simulink model "gm_parallel_lht"  (R2019b)
settings: Solver=FixedStepDiscrete  StartTime=0.0  StopTime=inf  RelTol=1e-3
undefined symbols (not defined in the file or in its folder): bt, height, width
libraries: hdlsllib x190, simulink x13, hdlmdlgenlib x7, dspsrcs4 x1
(part 14 of 18)

== system gm_parallel_lht/Parallel LHT/Parallel LHT Accumulator/Accumulator with Switches/Accumulator_instance150/Block RAM/Simple Dual Port RAM ==
  wr_data : Inport  OutDataTypeStr=fixdt(0, 11, 0)  PortDimensions=1  SampleTime=6.66666666666667e-09
  wr_addr : Inport  Port=2  OutDataTypeStr=fixdt(0, 11, 0)  PortDimensions=1  SampleTime=6.66666666666667e-09
  wr_en : Inport  Port=3  OutDataTypeStr=boolean  PortDimensions=1  SampleTime=6.66666666666667e-09
  rd_addr : Inport  Port=4  OutDataTypeStr=fixdt(0, 11, 0)  PortDimensions=1  SampleTime=6.66666666666667e-09
  Simple Dual Port RAM : hdlsllib/HDL RAMs/Simple Dual Port RAM  ram_size=ceil(log2(maxRho*2))
      settings: SourceProductName=Simulink  SourceProductBaseCode=SL
  rd_data : Outport
  wires:
  rd_addr/1 -> Simple Dual Port RAM/4
  wr_en/1 -> Simple Dual Port RAM/3
  wr_addr/1 -> Simple Dual Port RAM/2
  wr_data/1 -> Simple Dual Port RAM/1
  Simple Dual Port RAM/1 -> rd_data/1

== system gm_parallel_lht/Parallel LHT/Parallel LHT Accumulator/Accumulator with Switches/Accumulator_instance151/Block RAM/Simple Dual Port RAM ==
  wr_data : Inport  OutDataTypeStr=fixdt(0, 11, 0)  PortDimensions=1  SampleTime=6.66666666666667e-09
  wr_addr : Inport  Port=2  OutDataTypeStr=fixdt(0, 11, 0)  PortDimensions=1  SampleTime=6.66666666666667e-09
  wr_en : Inport  Port=3  OutDataTypeStr=boolean  PortDimensions=1  SampleTime=6.66666666666667e-09
  rd_addr : Inport  Port=4  OutDataTypeStr=fixdt(0, 11, 0)  PortDimensions=1  SampleTime=6.66666666666667e-09
  Simple Dual Port RAM : hdlsllib/HDL RAMs/Simple Dual Port RAM  ram_size=ceil(log2(maxRho*2))
      settings: SourceProductName=Simulink  SourceProductBaseCode=SL
  rd_data : Outport
  wires:
  rd_addr/1 -> Simple Dual Port RAM/4
  wr_en/1 -> Simple Dual Port RAM/3
  wr_addr/1 -> Simple Dual Port RAM/2
  wr_data/1 -> Simple Dual Port RAM/1
  Simple Dual Port RAM/1 -> rd_data/1

== system gm_parallel_lht/Parallel LHT/Parallel LHT Accumulator/Accumulator with Switches/Accumulator_instance152/Block RAM/Simple Dual Port RAM ==
  wr_data : Inport  OutDataTypeStr=fixdt(0, 11, 0)  PortDimensions=1  SampleTime=6.66666666666667e-09
  wr_addr : Inport  Port=2  OutDataTypeStr=fixdt(0, 11, 0)  PortDimensions=1  SampleTime=6.66666666666667e-09
  wr_en : Inport  Port=3  OutDataTypeStr=boolean  PortDimensions=1  SampleTime=6.66666666666667e-09
  rd_addr : Inport  Port=4  OutDataTypeStr=fixdt(0, 11, 0)  PortDimensions=1  SampleTime=6.66666666666667e-09
  Simple Dual Port RAM : hdlsllib/HDL RAMs/Simple Dual Port RAM  ram_size=ceil(log2(maxRho*2))
      settings: SourceProductName=Simulink  SourceProductBaseCode=SL
  rd_data : Outport
  wires:
  rd_addr/1 -> Simple Dual Port RAM/4
  wr_en/1 -> Simple Dual Port RAM/3
  wr_addr/1 -> Simple Dual Port RAM/2
  wr_data/1 -> Simple Dual Port RAM/1
  Simple Dual Port RAM/1 -> rd_data/1

== system gm_parallel_lht/Parallel LHT/Parallel LHT Accumulator/Accumulator with Switches/Accumulator_instance153/Block RAM/Simple Dual Port RAM ==
  wr_data : Inport  OutDataTypeStr=fixdt(0, 11, 0)  PortDimensions=1  SampleTime=6.66666666666667e-09
  wr_addr : Inport  Port=2  OutDataTypeStr=fixdt(0, 11, 0)  PortDimensions=1  SampleTime=6.66666666666667e-09
  wr_en : Inport  Port=3  OutDataTypeStr=boolean  PortDimensions=1  SampleTime=6.66666666666667e-09
  rd_addr : Inport  Port=4  OutDataTypeStr=fixdt(0, 11, 0)  PortDimensions=1  SampleTime=6.66666666666667e-09
  Simple Dual Port RAM : hdlsllib/HDL RAMs/Simple Dual Port RAM  ram_size=ceil(log2(maxRho*2))
      settings: SourceProductName=Simulink  SourceProductBaseCode=SL
  rd_data : Outport
  wires:
  rd_addr/1 -> Simple Dual Port RAM/4
  wr_en/1 -> Simple Dual Port RAM/3
  wr_addr/1 -> Simple Dual Port RAM/2
  wr_data/1 -> Simple Dual Port RAM/1
  Simple Dual Port RAM/1 -> rd_data/1

== system gm_parallel_lht/Parallel LHT/Parallel LHT Accumulator/Accumulator with Switches/Accumulator_instance154/Block RAM/Simple Dual Port RAM ==
  wr_data : Inport  OutDataTypeStr=fixdt(0, 11, 0)  PortDimensions=1  SampleTime=6.66666666666667e-09
  wr_addr : Inport  Port=2  OutDataTypeStr=fixdt(0, 11, 0)  PortDimensions=1  SampleTime=6.66666666666667e-09
  wr_en : Inport  Port=3  OutDataTypeStr=boolean  PortDimensions=1  SampleTime=6.66666666666667e-09
  rd_addr : Inport  Port=4  OutDataTypeStr=fixdt(0, 11, 0)  PortDimensions=1  SampleTime=6.66666666666667e-09
  Simple Dual Port RAM : hdlsllib/HDL RAMs/Simple Dual Port RAM  ram_size=ceil(log2(maxRho*2))
      settings: SourceProductName=Simulink  SourceProductBaseCode=SL
  rd_data : Outport
  wires:
  rd_addr/1 -> Simple Dual Port RAM/4
  wr_en/1 -> Simple Dual Port RAM/3
  wr_addr/1 -> Simple Dual Port RAM/2
  wr_data/1 -> Simple Dual Port RAM/1
  Simple Dual Port RAM/1 -> rd_data/1

== system gm_parallel_lht/Parallel LHT/Parallel LHT Accumulator/Accumulator with Switches/Accumulator_instance155/Block RAM/Simple Dual Port RAM ==
  wr_data : Inport  OutDataTypeStr=fixdt(0, 11, 0)  PortDimensions=1  SampleTime=6.66666666666667e-09
  wr_addr : Inport  Port=2  OutDataTypeStr=fixdt(0, 11, 0)  PortDimensions=1  SampleTime=6.66666666666667e-09
  wr_en : Inport  Port=3  OutDataTypeStr=boolean  PortDimensions=1  SampleTime=6.66666666666667e-09
  rd_addr : Inport  Port=4  OutDataTypeStr=fixdt(0, 11, 0)  PortDimensions=1  SampleTime=6.66666666666667e-09
  Simple Dual Port RAM : hdlsllib/HDL RAMs/Simple Dual Port RAM  ram_size=ceil(log2(maxRho*2))
      settings: SourceProductName=Simulink  SourceProductBaseCode=SL
  rd_data : Outport
  wires:
  rd_addr/1 -> Simple Dual Port RAM/4
  wr_en/1 -> Simple Dual Port RAM/3
  wr_addr/1 -> Simple Dual Port RAM/2
  wr_data/1 -> Simple Dual Port RAM/1
  Simple Dual Port RAM/1 -> rd_data/1

== system gm_parallel_lht/Parallel LHT/Parallel LHT Accumulator/Accumulator with Switches/Accumulator_instance156/Block RAM/Simple Dual Port RAM ==
  wr_data : Inport  OutDataTypeStr=fixdt(0, 11, 0)  PortDimensions=1  SampleTime=6.66666666666667e-09
  wr_addr : Inport  Port=2  OutDataTypeStr=fixdt(0, 11, 0)  PortDimensions=1  SampleTime=6.66666666666667e-09
  wr_en : Inport  Port=3  OutDataTypeStr=boolean  PortDimensions=1  SampleTime=6.66666666666667e-09
  rd_addr : Inport  Port=4  OutDataTypeStr=fixdt(0, 11, 0)  PortDimensions=1  SampleTime=6.66666666666667e-09
  Simple Dual Port RAM : hdlsllib/HDL RAMs/Simple Dual Port RAM  ram_size=ceil(log2(maxRho*2))
      settings: SourceProductName=Simulink  SourceProductBaseCode=SL
  rd_data : Outport
  wires:
  rd_addr/1 -> Simple Dual Port RAM/4
  wr_en/1 -> Simple Dual Port RAM/3
  wr_addr/1 -> Simple Dual Port RAM/2
  wr_data/1 -> Simple Dual Port RAM/1
  Simple Dual Port RAM/1 -> rd_data/1

== system gm_parallel_lht/Parallel LHT/Parallel LHT Accumulator/Accumulator with Switches/Accumulator_instance157/Block RAM/Simple Dual Port RAM ==
  wr_data : Inport  OutDataTypeStr=fixdt(0, 11, 0)  PortDimensions=1  SampleTime=6.66666666666667e-09
  wr_addr : Inport  Port=2  OutDataTypeStr=fixdt(0, 11, 0)  PortDimensions=1  SampleTime=6.66666666666667e-09
  wr_en : Inport  Port=3  OutDataTypeStr=boolean  PortDimensions=1  SampleTime=6.66666666666667e-09
  rd_addr : Inport  Port=4  OutDataTypeStr=fixdt(0, 11, 0)  PortDimensions=1  SampleTime=6.66666666666667e-09
  Simple Dual Port RAM : hdlsllib/HDL RAMs/Simple Dual Port RAM  ram_size=ceil(log2(maxRho*2))
      settings: SourceProductName=Simulink  SourceProductBaseCode=SL
  rd_data : Outport
  wires:
  rd_addr/1 -> Simple Dual Port RAM/4
  wr_en/1 -> Simple Dual Port RAM/3
  wr_addr/1 -> Simple Dual Port RAM/2
  wr_data/1 -> Simple Dual Port RAM/1
  Simple Dual Port RAM/1 -> rd_data/1

== system gm_parallel_lht/Parallel LHT/Parallel LHT Accumulator/Accumulator with Switches/Accumulator_instance158/Block RAM/Simple Dual Port RAM ==
  wr_data : Inport  OutDataTypeStr=fixdt(0, 11, 0)  PortDimensions=1  SampleTime=6.66666666666667e-09
  wr_addr : Inport  Port=2  OutDataTypeStr=fixdt(0, 11, 0)  PortDimensions=1  SampleTime=6.66666666666667e-09
  wr_en : Inport  Port=3  OutDataTypeStr=boolean  PortDimensions=1  SampleTime=6.66666666666667e-09
  rd_addr : Inport  Port=4  OutDataTypeStr=fixdt(0, 11, 0)  PortDimensions=1  SampleTime=6.66666666666667e-09
  Simple Dual Port RAM : hdlsllib/HDL RAMs/Simple Dual Port RAM  ram_size=ceil(log2(maxRho*2))
      settings: SourceProductName=Simulink  SourceProductBaseCode=SL
  rd_data : Outport
  wires:
  rd_addr/1 -> Simple Dual Port RAM/4
  wr_en/1 -> Simple Dual Port RAM/3
  wr_addr/1 -> Simple Dual Port RAM/2
  wr_data/1 -> Simple Dual Port RAM/1
  Simple Dual Port RAM/1 -> rd_data/1

== system gm_parallel_lht/Parallel LHT/Parallel LHT Accumulator/Accumulator with Switches/Accumulator_instance159/Block RAM/Simple Dual Port RAM ==
  wr_data : Inport  OutDataTypeStr=fixdt(0, 11, 0)  PortDimensions=1  SampleTime=6.66666666666667e-09
  wr_addr : Inport  Port=2  OutDataTypeStr=fixdt(0, 11, 0)  PortDimensions=1  SampleTime=6.66666666666667e-09
  wr_en : Inport  Port=3  OutDataTypeStr=boolean  PortDimensions=1  SampleTime=6.66666666666667e-09
  rd_addr : Inport  Port=4  OutDataTypeStr=fixdt(0, 11, 0)  PortDimensions=1  SampleTime=6.66666666666667e-09
  Simple Dual Port RAM : hdlsllib/HDL RAMs/Simple Dual Port RAM  ram_size=ceil(log2(maxRho*2))
      settings: SourceProductName=Simulink  SourceProductBaseCode=SL
  rd_data : Outport
  wires:
  rd_addr/1 -> Simple Dual Port RAM/4
  wr_en/1 -> Simple Dual Port RAM/3
  wr_addr/1 -> Simple Dual Port RAM/2
  wr_data/1 -> Simple Dual Port RAM/1
  Simple Dual Port RAM/1 -> rd_data/1

== system gm_parallel_lht/Parallel LHT/Parallel LHT Accumulator/Accumulator with Switches/Accumulator_instance16/Block RAM/Simple Dual Port RAM ==
  wr_data : Inport  OutDataTypeStr=fixdt(0, 11, 0)  PortDimensions=1  SampleTime=6.66666666666667e-09
  wr_addr : Inport  Port=2  OutDataTypeStr=fixdt(0, 11, 0)  PortDimensions=1  SampleTime=6.66666666666667e-09
  wr_en : Inport  Port=3  OutDataTypeStr=boolean  PortDimensions=1  SampleTime=6.66666666666667e-09
  rd_addr : Inport  Port=4  OutDataTypeStr=fixdt(0, 11, 0)  PortDimensions=1  SampleTime=6.66666666666667e-09
  Simple Dual Port RAM : hdlsllib/HDL RAMs/Simple Dual Port RAM  ram_size=ceil(log2(maxRho*2))
      settings: SourceProductName=Simulink  SourceProductBaseCode=SL
  rd_data : Outport
  wires:
  rd_addr/1 -> Simple Dual Port RAM/4
  wr_en/1 -> Simple Dual Port RAM/3
  wr_addr/1 -> Simple Dual Port RAM/2
  wr_data/1 -> Simple Dual Port RAM/1
  Simple Dual Port RAM/1 -> rd_data/1

== system gm_parallel_lht/Parallel LHT/Parallel LHT Accumulator/Accumulator with Switches/Accumulator_instance160/Block RAM/Simple Dual Port RAM ==
  wr_data : Inport  OutDataTypeStr=fixdt(0, 11, 0)  PortDimensions=1  SampleTime=6.66666666666667e-09
  wr_addr : Inport  Port=2  OutDataTypeStr=fixdt(0, 11, 0)  PortDimensions=1  SampleTime=6.66666666666667e-09
  wr_en : Inport  Port=3  OutDataTypeStr=boolean  PortDimensions=1  SampleTime=6.66666666666667e-09
  rd_addr : Inport  Port=4  OutDataTypeStr=fixdt(0, 11, 0)  PortDimensions=1  SampleTime=6.66666666666667e-09
  Simple Dual Port RAM : hdlsllib/HDL RAMs/Simple Dual Port RAM  ram_size=ceil(log2(maxRho*2))
      settings: SourceProductName=Simulink  SourceProductBaseCode=SL
  rd_data : Outport
  wires:
  rd_addr/1 -> Simple Dual Port RAM/4
  wr_en/1 -> Simple Dual Port RAM/3
  wr_addr/1 -> Simple Dual Port RAM/2
  wr_data/1 -> Simple Dual Port RAM/1
  Simple Dual Port RAM/1 -> rd_data/1

== system gm_parallel_lht/Parallel LHT/Parallel LHT Accumulator/Accumulator with Switches/Accumulator_instance161/Block RAM/Simple Dual Port RAM ==
  wr_data : Inport  OutDataTypeStr=fixdt(0, 11, 0)  PortDimensions=1  SampleTime=6.66666666666667e-09
  wr_addr : Inport  Port=2  OutDataTypeStr=fixdt(0, 11, 0)  PortDimensions=1  SampleTime=6.66666666666667e-09
  wr_en : Inport  Port=3  OutDataTypeStr=boolean  PortDimensions=1  SampleTime=6.66666666666667e-09
  rd_addr : Inport  Port=4  OutDataTypeStr=fixdt(0, 11, 0)  PortDimensions=1  SampleTime=6.66666666666667e-09
  Simple Dual Port RAM : hdlsllib/HDL RAMs/Simple Dual Port RAM  ram_size=ceil(log2(maxRho*2))
      settings: SourceProductName=Simulink  SourceProductBaseCode=SL
  rd_data : Outport
  wires:
  rd_addr/1 -> Simple Dual Port RAM/4
  wr_en/1 -> Simple Dual Port RAM/3
  wr_addr/1 -> Simple Dual Port RAM/2
  wr_data/1 -> Simple Dual Port RAM/1
  Simple Dual Port RAM/1 -> rd_data/1

== system gm_parallel_lht/Parallel LHT/Parallel LHT Accumulator/Accumulator with Switches/Accumulator_instance162/Block RAM/Simple Dual Port RAM ==
  wr_data : Inport  OutDataTypeStr=fixdt(0, 11, 0)  PortDimensions=1  SampleTime=6.66666666666667e-09
  wr_addr : Inport  Port=2  OutDataTypeStr=fixdt(0, 11, 0)  PortDimensions=1  SampleTime=6.66666666666667e-09
  wr_en : Inport  Port=3  OutDataTypeStr=boolean  PortDimensions=1  SampleTime=6.66666666666667e-09
  rd_addr : Inport  Port=4  OutDataTypeStr=fixdt(0, 11, 0)  PortDimensions=1  SampleTime=6.66666666666667e-09
  Simple Dual Port RAM : hdlsllib/HDL RAMs/Simple Dual Port RAM  ram_size=ceil(log2(maxRho*2))
      settings: SourceProductName=Simulink  SourceProductBaseCode=SL
  rd_data : Outport
  wires:
  rd_addr/1 -> Simple Dual Port RAM/4
  wr_en/1 -> Simple Dual Port RAM/3
  wr_addr/1 -> Simple Dual Port RAM/2
  wr_data/1 -> Simple Dual Port RAM/1
  Simple Dual Port RAM/1 -> rd_data/1

== system gm_parallel_lht/Parallel LHT/Parallel LHT Accumulator/Accumulator with Switches/Accumulator_instance163/Block RAM/Simple Dual Port RAM ==
  wr_data : Inport  OutDataTypeStr=fixdt(0, 11, 0)  PortDimensions=1  SampleTime=6.66666666666667e-09
  wr_addr : Inport  Port=2  OutDataTypeStr=fixdt(0, 11, 0)  PortDimensions=1  SampleTime=6.66666666666667e-09
  wr_en : Inport  Port=3  OutDataTypeStr=boolean  PortDimensions=1  SampleTime=6.66666666666667e-09
  rd_addr : Inport  Port=4  OutDataTypeStr=fixdt(0, 11, 0)  PortDimensions=1  SampleTime=6.66666666666667e-09
  Simple Dual Port RAM : hdlsllib/HDL RAMs/Simple Dual Port RAM  ram_size=ceil(log2(maxRho*2))
      settings: SourceProductName=Simulink  SourceProductBaseCode=SL
  rd_data : Outport
  wires:
  rd_addr/1 -> Simple Dual Port RAM/4
  wr_en/1 -> Simple Dual Port RAM/3
  wr_addr/1 -> Simple Dual Port RAM/2
  wr_data/1 -> Simple Dual Port RAM/1
  Simple Dual Port RAM/1 -> rd_data/1

== system gm_parallel_lht/Parallel LHT/Parallel LHT Accumulator/Accumulator with Switches/Accumulator_instance164/Block RAM/Simple Dual Port RAM ==
  wr_data : Inport  OutDataTypeStr=fixdt(0, 11, 0)  PortDimensions=1  SampleTime=6.66666666666667e-09
  wr_addr : Inport  Port=2  OutDataTypeStr=fixdt(0, 11, 0)  PortDimensions=1  SampleTime=6.66666666666667e-09
  wr_en : Inport  Port=3  OutDataTypeStr=boolean  PortDimensions=1  SampleTime=6.66666666666667e-09
  rd_addr : Inport  Port=4  OutDataTypeStr=fixdt(0, 11, 0)  PortDimensions=1  SampleTime=6.66666666666667e-09
  Simple Dual Port RAM : hdlsllib/HDL RAMs/Simple Dual Port RAM  ram_size=ceil(log2(maxRho*2))
      settings: SourceProductName=Simulink  SourceProductBaseCode=SL
  rd_data : Outport
  wires:
  rd_addr/1 -> Simple Dual Port RAM/4
  wr_en/1 -> Simple Dual Port RAM/3
  wr_addr/1 -> Simple Dual Port RAM/2
  wr_data/1 -> Simple Dual Port RAM/1
  Simple Dual Port RAM/1 -> rd_data/1

== system gm_parallel_lht/Parallel LHT/Parallel LHT Accumulator/Accumulator with Switches/Accumulator_instance165/Block RAM/Simple Dual Port RAM ==
  wr_data : Inport  OutDataTypeStr=fixdt(0, 11, 0)  PortDimensions=1  SampleTime=6.66666666666667e-09
  wr_addr : Inport  Port=2  OutDataTypeStr=fixdt(0, 11, 0)  PortDimensions=1  SampleTime=6.66666666666667e-09
  wr_en : Inport  Port=3  OutDataTypeStr=boolean  PortDimensions=1  SampleTime=6.66666666666667e-09
  rd_addr : Inport  Port=4  OutDataTypeStr=fixdt(0, 11, 0)  PortDimensions=1  SampleTime=6.66666666666667e-09
  Simple Dual Port RAM : hdlsllib/HDL RAMs/Simple Dual Port RAM  ram_size=ceil(log2(maxRho*2))
      settings: SourceProductName=Simulink  SourceProductBaseCode=SL
  rd_data : Outport
  wires:
  rd_addr/1 -> Simple Dual Port RAM/4
  wr_en/1 -> Simple Dual Port RAM/3
  wr_addr/1 -> Simple Dual Port RAM/2
  wr_data/1 -> Simple Dual Port RAM/1
  Simple Dual Port RAM/1 -> rd_data/1

== system gm_parallel_lht/Parallel LHT/Parallel LHT Accumulator/Accumulator with Switches/Accumulator_instance166/Block RAM/Simple Dual Port RAM ==
  wr_data : Inport  OutDataTypeStr=fixdt(0, 11, 0)  PortDimensions=1  SampleTime=6.66666666666667e-09
  wr_addr : Inport  Port=2  OutDataTypeStr=fixdt(0, 11, 0)  PortDimensions=1  SampleTime=6.66666666666667e-09
  wr_en : Inport  Port=3  OutDataTypeStr=boolean  PortDimensions=1  SampleTime=6.66666666666667e-09
  rd_addr : Inport  Port=4  OutDataTypeStr=fixdt(0, 11, 0)  PortDimensions=1  SampleTime=6.66666666666667e-09
  Simple Dual Port RAM : hdlsllib/HDL RAMs/Simple Dual Port RAM  ram_size=ceil(log2(maxRho*2))
      settings: SourceProductName=Simulink  SourceProductBaseCode=SL
  rd_data : Outport
  wires:
  rd_addr/1 -> Simple Dual Port RAM/4
  wr_en/1 -> Simple Dual Port RAM/3
  wr_addr/1 -> Simple Dual Port RAM/2
  wr_data/1 -> Simple Dual Port RAM/1
  Simple Dual Port RAM/1 -> rd_data/1

== system gm_parallel_lht/Parallel LHT/Parallel LHT Accumulator/Accumulator with Switches/Accumulator_instance167/Block RAM/Simple Dual Port RAM ==
  wr_data : Inport  OutDataTypeStr=fixdt(0, 11, 0)  PortDimensions=1  SampleTime=6.66666666666667e-09
  wr_addr : Inport  Port=2  OutDataTypeStr=fixdt(0, 11, 0)  PortDimensions=1  SampleTime=6.66666666666667e-09
  wr_en : Inport  Port=3  OutDataTypeStr=boolean  PortDimensions=1  SampleTime=6.66666666666667e-09
  rd_addr : Inport  Port=4  OutDataTypeStr=fixdt(0, 11, 0)  PortDimensions=1  SampleTime=6.66666666666667e-09
  Simple Dual Port RAM : hdlsllib/HDL RAMs/Simple Dual Port RAM  ram_size=ceil(log2(maxRho*2))
      settings: SourceProductName=Simulink  SourceProductBaseCode=SL
  rd_data : Outport
  wires:
  rd_addr/1 -> Simple Dual Port RAM/4
  wr_en/1 -> Simple Dual Port RAM/3
  wr_addr/1 -> Simple Dual Port RAM/2
  wr_data/1 -> Simple Dual Port RAM/1
  Simple Dual Port RAM/1 -> rd_data/1

== system gm_parallel_lht/Parallel LHT/Parallel LHT Accumulator/Accumulator with Switches/Accumulator_instance168/Block RAM/Simple Dual Port RAM ==
  wr_data : Inport  OutDataTypeStr=fixdt(0, 11, 0)  PortDimensions=1  SampleTime=6.66666666666667e-09
  wr_addr : Inport  Port=2  OutDataTypeStr=fixdt(0, 11, 0)  PortDimensions=1  SampleTime=6.66666666666667e-09
  wr_en : Inport  Port=3  OutDataTypeStr=boolean  PortDimensions=1  SampleTime=6.66666666666667e-09
  rd_addr : Inport  Port=4  OutDataTypeStr=fixdt(0, 11, 0)  PortDimensions=1  SampleTime=6.66666666666667e-09
  Simple Dual Port RAM : hdlsllib/HDL RAMs/Simple Dual Port RAM  ram_size=ceil(log2(maxRho*2))
      settings: SourceProductName=Simulink  SourceProductBaseCode=SL
  rd_data : Outport
  wires:
  rd_addr/1 -> Simple Dual Port RAM/4
  wr_en/1 -> Simple Dual Port RAM/3
  wr_addr/1 -> Simple Dual Port RAM/2
  wr_data/1 -> Simple Dual Port RAM/1
  Simple Dual Port RAM/1 -> rd_data/1

== system gm_parallel_lht/Parallel LHT/Parallel LHT Accumulator/Accumulator with Switches/Accumulator_instance169/Block RAM/Simple Dual Port RAM ==
  wr_data : Inport  OutDataTypeStr=fixdt(0, 11, 0)  PortDimensions=1  SampleTime=6.66666666666667e-09
  wr_addr : Inport  Port=2  OutDataTypeStr=fixdt(0, 11, 0)  PortDimensions=1  SampleTime=6.66666666666667e-09
  wr_en : Inport  Port=3  OutDataTypeStr=boolean  PortDimensions=1  SampleTime=6.66666666666667e-09
  rd_addr : Inport  Port=4  OutDataTypeStr=fixdt(0, 11, 0)  PortDimensions=1  SampleTime=6.66666666666667e-09
  Simple Dual Port RAM : hdlsllib/HDL RAMs/Simple Dual Port RAM  ram_size=ceil(log2(maxRho*2))
      settings: SourceProductName=Simulink  SourceProductBaseCode=SL
  rd_data : Outport
  wires:
  rd_addr/1 -> Simple Dual Port RAM/4
  wr_en/1 -> Simple Dual Port RAM/3
  wr_addr/1 -> Simple Dual Port RAM/2
  wr_data/1 -> Simple Dual Port RAM/1
  Simple Dual Port RAM/1 -> rd_data/1

== system gm_parallel_lht/Parallel LHT/Parallel LHT Accumulator/Accumulator with Switches/Accumulator_instance17/Block RAM/Simple Dual Port RAM ==
  wr_data : Inport  OutDataTypeStr=fixdt(0, 11, 0)  PortDimensions=1  SampleTime=6.66666666666667e-09
  wr_addr : Inport  Port=2  OutDataTypeStr=fixdt(0, 11, 0)  PortDimensions=1  SampleTime=6.66666666666667e-09
  wr_en : Inport  Port=3  OutDataTypeStr=boolean  PortDimensions=1  SampleTime=6.66666666666667e-09
  rd_addr : Inport  Port=4  OutDataTypeStr=fixdt(0, 11, 0)  PortDimensions=1  SampleTime=6.66666666666667e-09
  Simple Dual Port RAM : hdlsllib/HDL RAMs/Simple Dual Port RAM  ram_size=ceil(log2(maxRho*2))
      settings: SourceProductName=Simulink  SourceProductBaseCode=SL
  rd_data : Outport
  wires:
  rd_addr/1 -> Simple Dual Port RAM/4
  wr_en/1 -> Simple Dual Port RAM/3
  wr_addr/1 -> Simple Dual Port RAM/2
  wr_data/1 -> Simple Dual Port RAM/1
  Simple Dual Port RAM/1 -> rd_data/1

== system gm_parallel_lht/Parallel LHT/Parallel LHT Accumulator/Accumulator with Switches/Accumulator_instance170/Block RAM/Simple Dual Port RAM ==
  wr_data : Inport  OutDataTypeStr=fixdt(0, 11, 0)  PortDimensions=1  SampleTime=6.66666666666667e-09
  wr_addr : Inport  Port=2  OutDataTypeStr=fixdt(0, 11, 0)  PortDimensions=1  SampleTime=6.66666666666667e-09
  wr_en : Inport  Port=3  OutDataTypeStr=boolean  PortDimensions=1  SampleTime=6.66666666666667e-09
  rd_addr : Inport  Port=4  OutDataTypeStr=fixdt(0, 11, 0)  PortDimensions=1  SampleTime=6.66666666666667e-09
  Simple Dual Port RAM : hdlsllib/HDL RAMs/Simple Dual Port RAM  ram_size=ceil(log2(maxRho*2))
      settings: SourceProductName=Simulink  SourceProductBaseCode=SL
  rd_data : Outport
  wires:
  rd_addr/1 -> Simple Dual Port RAM/4
  wr_en/1 -> Simple Dual Port RAM/3
  wr_addr/1 -> Simple Dual Port RAM/2
  wr_data/1 -> Simple Dual Port RAM/1
  Simple Dual Port RAM/1 -> rd_data/1

== system gm_parallel_lht/Parallel LHT/Parallel LHT Accumulator/Accumulator with Switches/Accumulator_instance171/Block RAM/Simple Dual Port RAM ==
  wr_data : Inport  OutDataTypeStr=fixdt(0, 11, 0)  PortDimensions=1  SampleTime=6.66666666666667e-09
  wr_addr : Inport  Port=2  OutDataTypeStr=fixdt(0, 11, 0)  PortDimensions=1  SampleTime=6.66666666666667e-09
  wr_en : Inport  Port=3  OutDataTypeStr=boolean  PortDimensions=1  SampleTime=6.66666666666667e-09
  rd_addr : Inport  Port=4  OutDataTypeStr=fixdt(0, 11, 0)  PortDimensions=1  SampleTime=6.66666666666667e-09
  Simple Dual Port RAM : hdlsllib/HDL RAMs/Simple Dual Port RAM  ram_size=ceil(log2(maxRho*2))
      settings: SourceProductName=Simulink  SourceProductBaseCode=SL
  rd_data : Outport
  wires:
  rd_addr/1 -> Simple Dual Port RAM/4
  wr_en/1 -> Simple Dual Port RAM/3
  wr_addr/1 -> Simple Dual Port RAM/2
  wr_data/1 -> Simple Dual Port RAM/1
  Simple Dual Port RAM/1 -> rd_data/1

== system gm_parallel_lht/Parallel LHT/Parallel LHT Accumulator/Accumulator with Switches/Accumulator_instance172/Block RAM/Simple Dual Port RAM ==
  wr_data : Inport  OutDataTypeStr=fixdt(0, 11, 0)  PortDimensions=1  SampleTime=6.66666666666667e-09
  wr_addr : Inport  Port=2  OutDataTypeStr=fixdt(0, 11, 0)  PortDimensions=1  SampleTime=6.66666666666667e-09
  wr_en : Inport  Port=3  OutDataTypeStr=boolean  PortDimensions=1  SampleTime=6.66666666666667e-09
  rd_addr : Inport  Port=4  OutDataTypeStr=fixdt(0, 11, 0)  PortDimensions=1  SampleTime=6.66666666666667e-09
  Simple Dual Port RAM : hdlsllib/HDL RAMs/Simple Dual Port RAM  ram_size=ceil(log2(maxRho*2))
      settings: SourceProductName=Simulink  SourceProductBaseCode=SL
  rd_data : Outport
  wires:
  rd_addr/1 -> Simple Dual Port RAM/4
  wr_en/1 -> Simple Dual Port RAM/3
  wr_addr/1 -> Simple Dual Port RAM/2
  wr_data/1 -> Simple Dual Port RAM/1
  Simple Dual Port RAM/1 -> rd_data/1

== system gm_parallel_lht/Parallel LHT/Parallel LHT Accumulator/Accumulator with Switches/Accumulator_instance173/Block RAM/Simple Dual Port RAM ==
  wr_data : Inport  OutDataTypeStr=fixdt(0, 11, 0)  PortDimensions=1  SampleTime=6.66666666666667e-09
  wr_addr : Inport  Port=2  OutDataTypeStr=fixdt(0, 11, 0)  PortDimensions=1  SampleTime=6.66666666666667e-09
  wr_en : Inport  Port=3  OutDataTypeStr=boolean  PortDimensions=1  SampleTime=6.66666666666667e-09
  rd_addr : Inport  Port=4  OutDataTypeStr=fixdt(0, 11, 0)  PortDimensions=1  SampleTime=6.66666666666667e-09
  Simple Dual Port RAM : hdlsllib/HDL RAMs/Simple Dual Port RAM  ram_size=ceil(log2(maxRho*2))
      settings: SourceProductName=Simulink  SourceProductBaseCode=SL
  rd_data : Outport
  wires:
  rd_addr/1 -> Simple Dual Port RAM/4
  wr_en/1 -> Simple Dual Port RAM/3
  wr_addr/1 -> Simple Dual Port RAM/2
  wr_data/1 -> Simple Dual Port RAM/1
  Simple Dual Port RAM/1 -> rd_data/1

== system gm_parallel_lht/Parallel LHT/Parallel LHT Accumulator/Accumulator with Switches/Accumulator_instance174/Block RAM/Simple Dual Port RAM ==
  wr_data : Inport  OutDataTypeStr=fixdt(0, 11, 0)  PortDimensions=1  SampleTime=6.66666666666667e-09
  wr_addr : Inport  Port=2  OutDataTypeStr=fixdt(0, 11, 0)  PortDimensions=1  SampleTime=6.66666666666667e-09
  wr_en : Inport  Port=3  OutDataTypeStr=boolean  PortDimensions=1  SampleTime=6.66666666666667e-09
  rd_addr : Inport  Port=4  OutDataTypeStr=fixdt(0, 11, 0)  PortDimensions=1  SampleTime=6.66666666666667e-09
  Simple Dual Port RAM : hdlsllib/HDL RAMs/Simple Dual Port RAM  ram_size=ceil(log2(maxRho*2))
      settings: SourceProductName=Simulink  SourceProductBaseCode=SL
  rd_data : Outport
  wires:
  rd_addr/1 -> Simple Dual Port RAM/4
  wr_en/1 -> Simple Dual Port RAM/3
  wr_addr/1 -> Simple Dual Port RAM/2
  wr_data/1 -> Simple Dual Port RAM/1
  Simple Dual Port RAM/1 -> rd_data/1

== system gm_parallel_lht/Parallel LHT/Parallel LHT Accumulator/Accumulator with Switches/Accumulator_instance175/Block RAM/Simple Dual Port RAM ==
  wr_data : Inport  OutDataTypeStr=fixdt(0, 11, 0)  PortDimensions=1  SampleTime=6.66666666666667e-09
  wr_addr : Inport  Port=2  OutDataTypeStr=fixdt(0, 11, 0)  PortDimensions=1  SampleTime=6.66666666666667e-09
  wr_en : Inport  Port=3  OutDataTypeStr=boolean  PortDimensions=1  SampleTime=6.66666666666667e-09
  rd_addr : Inport  Port=4  OutDataTypeStr=fixdt(0, 11, 0)  PortDimensions=1  SampleTime=6.66666666666667e-09
  Simple Dual Port RAM : hdlsllib/HDL RAMs/Simple Dual Port RAM  ram_size=ceil(log2(maxRho*2))
      settings: SourceProductName=Simulink  SourceProductBaseCode=SL
  rd_data : Outport
  wires:
  rd_addr/1 -> Simple Dual Port RAM/4
  wr_en/1 -> Simple Dual Port RAM/3
  wr_addr/1 -> Simple Dual Port RAM/2
  wr_data/1 -> Simple Dual Port RAM/1
  Simple Dual Port RAM/1 -> rd_data/1

== system gm_parallel_lht/Parallel LHT/Parallel LHT Accumulator/Accumulator with Switches/Accumulator_instance176/Block RAM/Simple Dual Port RAM ==
  wr_data : Inport  OutDataTypeStr=fixdt(0, 11, 0)  PortDimensions=1  SampleTime=6.66666666666667e-09
  wr_addr : Inport  Port=2  OutDataTypeStr=fixdt(0, 11, 0)  PortDimensions=1  SampleTime=6.66666666666667e-09
  wr_en : Inport  Port=3  OutDataTypeStr=boolean  PortDimensions=1  SampleTime=6.66666666666667e-09
  rd_addr : Inport  Port=4  OutDataTypeStr=fixdt(0, 11, 0)  PortDimensions=1  SampleTime=6.66666666666667e-09
  Simple Dual Port RAM : hdlsllib/HDL RAMs/Simple Dual Port RAM  ram_size=ceil(log2(maxRho*2))
      settings: SourceProductName=Simulink  SourceProductBaseCode=SL
  rd_data : Outport
  wires:
  rd_addr/1 -> Simple Dual Port RAM/4
  wr_en/1 -> Simple Dual Port RAM/3
  wr_addr/1 -> Simple Dual Port RAM/2
  wr_data/1 -> Simple Dual Port RAM/1
  Simple Dual Port RAM/1 -> rd_data/1

== system gm_parallel_lht/Parallel LHT/Parallel LHT Accumulator/Accumulator with Switches/Accumulator_instance177/Block RAM/Simple Dual Port RAM ==
  wr_data : Inport  OutDataTypeStr=fixdt(0, 11, 0)  PortDimensions=1  SampleTime=6.66666666666667e-09
  wr_addr : Inport  Port=2  OutDataTypeStr=fixdt(0, 11, 0)  PortDimensions=1  SampleTime=6.66666666666667e-09
  wr_en : Inport  Port=3  OutDataTypeStr=boolean  PortDimensions=1  SampleTime=6.66666666666667e-09
  rd_addr : Inport  Port=4  OutDataTypeStr=fixdt(0, 11, 0)  PortDimensions=1  SampleTime=6.66666666666667e-09
  Simple Dual Port RAM : hdlsllib/HDL RAMs/Simple Dual Port RAM  ram_size=ceil(log2(maxRho*2))
      settings: SourceProductName=Simulink  SourceProductBaseCode=SL
  rd_data : Outport
  wires:
  rd_addr/1 -> Simple Dual Port RAM/4
  wr_en/1 -> Simple Dual Port RAM/3
  wr_addr/1 -> Simple Dual Port RAM/2
  wr_data/1 -> Simple Dual Port RAM/1
  Simple Dual Port RAM/1 -> rd_data/1

== system gm_parallel_lht/Parallel LHT/Parallel LHT Accumulator/Accumulator with Switches/Accumulator_instance178/Block RAM/Simple Dual Port RAM ==
  wr_data : Inport  OutDataTypeStr=fixdt(0, 11, 0)  PortDimensions=1  SampleTime=6.66666666666667e-09
  wr_addr : Inport  Port=2  OutDataTypeStr=fixdt(0, 11, 0)  PortDimensions=1  SampleTime=6.66666666666667e-09
  wr_en : Inport  Port=3  OutDataTypeStr=boolean  PortDimensions=1  SampleTime=6.66666666666667e-09
  rd_addr : Inport  Port=4  OutDataTypeStr=fixdt(0, 11, 0)  PortDimensions=1  SampleTime=6.66666666666667e-09
  Simple Dual Port RAM : hdlsllib/HDL RAMs/Simple Dual Port RAM  ram_size=ceil(log2(maxRho*2))
      settings: SourceProductName=Simulink  SourceProductBaseCode=SL
  rd_data : Outport
  wires:
  rd_addr/1 -> Simple Dual Port RAM/4
  wr_en/1 -> Simple Dual Port RAM/3
  wr_addr/1 -> Simple Dual Port RAM/2
  wr_data/1 -> Simple Dual Port RAM/1
  Simple Dual Port RAM/1 -> rd_data/1

== system gm_parallel_lht/Parallel LHT/Parallel LHT Accumulator/Accumulator with Switches/Accumulator_instance179/Block RAM/Simple Dual Port RAM ==
  wr_data : Inport  OutDataTypeStr=fixdt(0, 11, 0)  PortDimensions=1  SampleTime=6.66666666666667e-09
  wr_addr : Inport  Port=2  OutDataTypeStr=fixdt(0, 11, 0)  PortDimensions=1  SampleTime=6.66666666666667e-09
  wr_en : Inport  Port=3  OutDataTypeStr=boolean  PortDimensions=1  SampleTime=6.66666666666667e-09
  rd_addr : Inport  Port=4  OutDataTypeStr=fixdt(0, 11, 0)  PortDimensions=1  SampleTime=6.66666666666667e-09
  Simple Dual Port RAM : hdlsllib/HDL RAMs/Simple Dual Port RAM  ram_size=ceil(log2(maxRho*2))
      settings: SourceProductName=Simulink  SourceProductBaseCode=SL
  rd_data : Outport
  wires:
  rd_addr/1 -> Simple Dual Port RAM/4
  wr_en/1 -> Simple Dual Port RAM/3
  wr_addr/1 -> Simple Dual Port RAM/2
  wr_data/1 -> Simple Dual Port RAM/1
  Simple Dual Port RAM/1 -> rd_data/1

== system gm_parallel_lht/Parallel LHT/Parallel LHT Accumulator/Accumulator with Switches/Accumulator_instance18/Block RAM/Simple Dual Port RAM ==
  wr_data : Inport  OutDataTypeStr=fixdt(0, 11, 0)  PortDimensions=1  SampleTime=6.66666666666667e-09
  wr_addr : Inport  Port=2  OutDataTypeStr=fixdt(0, 11, 0)  PortDimensions=1  SampleTime=6.66666666666667e-09
  wr_en : Inport  Port=3  OutDataTypeStr=boolean  PortDimensions=1  SampleTime=6.66666666666667e-09
  rd_addr : Inport  Port=4  OutDataTypeStr=fixdt(0, 11, 0)  PortDimensions=1  SampleTime=6.66666666666667e-09
  Simple Dual Port RAM : hdlsllib/HDL RAMs/Simple Dual Port RAM  ram_size=ceil(log2(maxRho*2))
      settings: SourceProductName=Simulink  SourceProductBaseCode=SL
  rd_data : Outport
  wires:
  rd_addr/1 -> Simple Dual Port RAM/4
  wr_en/1 -> Simple Dual Port RAM/3
  wr_addr/1 -> Simple Dual Port RAM/2
  wr_data/1 -> Simple Dual Port RAM/1
  Simple Dual Port RAM/1 -> rd_data/1

== system gm_parallel_lht/Parallel LHT/Parallel LHT Accumulator/Accumulator with Switches/Accumulator_instance180/Block RAM/Simple Dual Port RAM ==
  wr_data : Inport  OutDataTypeStr=fixdt(0, 11, 0)  PortDimensions=1  SampleTime=6.66666666666667e-09
  wr_addr : Inport  Port=2  OutDataTypeStr=fixdt(0, 11, 0)  PortDimensions=1  SampleTime=6.66666666666667e-09
  wr_en : Inport  Port=3  OutDataTypeStr=boolean  PortDimensions=1  SampleTime=6.66666666666667e-09
  rd_addr : Inport  Port=4  OutDataTypeStr=fixdt(0, 11, 0)  PortDimensions=1  SampleTime=6.66666666666667e-09
  Simple Dual Port RAM : hdlsllib/HDL RAMs/Simple Dual Port RAM  ram_size=ceil(log2(maxRho*2))
      settings: SourceProductName=Simulink  SourceProductBaseCode=SL
  rd_data : Outport
  wires:
  rd_addr/1 -> Simple Dual Port RAM/4
  wr_en/1 -> Simple Dual Port RAM/3
  wr_addr/1 -> Simple Dual Port RAM/2
  wr_data/1 -> Simple Dual Port RAM/1
  Simple Dual Port RAM/1 -> rd_data/1

== system gm_parallel_lht/Parallel LHT/Parallel LHT Accumulator/Accumulator with Switches/Accumulator_instance19/Block RAM/Simple Dual Port RAM ==
  wr_data : Inport  OutDataTypeStr=fixdt(0, 11, 0)  PortDimensions=1  SampleTime=6.66666666666667e-09
  wr_addr : Inport  Port=2  OutDataTypeStr=fixdt(0, 11, 0)  PortDimensions=1  SampleTime=6.66666666666667e-09
  wr_en : Inport  Port=3  OutDataTypeStr=boolean  PortDimensions=1  SampleTime=6.66666666666667e-09
  rd_addr : Inport  Port=4  OutDataTypeStr=fixdt(0, 11, 0)  PortDimensions=1  SampleTime=6.66666666666667e-09
  Simple Dual Port RAM : hdlsllib/HDL RAMs/Simple Dual Port RAM  ram_size=ceil(log2(maxRho*2))
      settings: SourceProductName=Simulink  SourceProductBaseCode=SL
  rd_data : Outport
  wires:
  rd_addr/1 -> Simple Dual Port RAM/4
  wr_en/1 -> Simple Dual Port RAM/3
  wr_addr/1 -> Simple Dual Port RAM/2
  wr_data/1 -> Simple Dual Port RAM/1
  Simple Dual Port RAM/1 -> rd_data/1

== system gm_parallel_lht/Parallel LHT/Parallel LHT Accumulator/Accumulator with Switches/Accumulator_instance2/Block RAM/Simple Dual Port RAM ==
  wr_data : Inport  OutDataTypeStr=fixdt(0, 11, 0)  PortDimensions=1  SampleTime=6.66666666666667e-09
  wr_addr : Inport  Port=2  OutDataTypeStr=fixdt(0, 11, 0)  PortDimensions=1  SampleTime=6.66666666666667e-09
  wr_en : Inport  Port=3  OutDataTypeStr=boolean  PortDimensions=1  SampleTime=6.66666666666667e-09
  rd_addr : Inport  Port=4  OutDataTypeStr=fixdt(0, 11, 0)  PortDimensions=1  SampleTime=6.66666666666667e-09
  Simple Dual Port RAM : hdlsllib/HDL RAMs/Simple Dual Port RAM  ram_size=ceil(log2(maxRho*2))
      settings: SourceProductName=Simulink  SourceProductBaseCode=SL
  rd_data : Outport
  wires:
  rd_addr/1 -> Simple Dual Port RAM/4
  wr_en/1 -> Simple Dual Port RAM/3
  wr_addr/1 -> Simple Dual Port RAM/2
  wr_data/1 -> Simple Dual Port RAM/1
  Simple Dual Port RAM/1 -> rd_data/1

== system gm_parallel_lht/Parallel LHT/Parallel LHT Accumulator/Accumulator with Switches/Accumulator_instance20/Block RAM/Simple Dual Port RAM ==
  wr_data : Inport  OutDataTypeStr=fixdt(0, 11, 0)  PortDimensions=1  SampleTime=6.66666666666667e-09
  wr_addr : Inport  Port=2  OutDataTypeStr=fixdt(0, 11, 0)  PortDimensions=1  SampleTime=6.66666666666667e-09
  wr_en : Inport  Port=3  OutDataTypeStr=boolean  PortDimensions=1  SampleTime=6.66666666666667e-09
  rd_addr : Inport  Port=4  OutDataTypeStr=fixdt(0, 11, 0)  PortDimensions=1  SampleTime=6.66666666666667e-09
  Simple Dual Port RAM : hdlsllib/HDL RAMs/Simple Dual Port RAM  ram_size=ceil(log2(maxRho*2))
      settings: SourceProductName=Simulink  SourceProductBaseCode=SL
  rd_data : Outport
  wires:
  rd_addr/1 -> Simple Dual Port RAM/4
  wr_en/1 -> Simple Dual Port RAM/3
  wr_addr/1 -> Simple Dual Port RAM/2
  wr_data/1 -> Simple Dual Port RAM/1
  Simple Dual Port RAM/1 -> rd_data/1

== system gm_parallel_lht/Parallel LHT/Parallel LHT Accumulator/Accumulator with Switches/Accumulator_instance21/Block RAM/Simple Dual Port RAM ==
  wr_data : Inport  OutDataTypeStr=fixdt(0, 11, 0)  PortDimensions=1  SampleTime=6.66666666666667e-09
  wr_addr : Inport  Port=2  OutDataTypeStr=fixdt(0, 11, 0)  PortDimensions=1  SampleTime=6.66666666666667e-09
  wr_en : Inport  Port=3  OutDataTypeStr=boolean  PortDimensions=1  SampleTime=6.66666666666667e-09
  rd_addr : Inport  Port=4  OutDataTypeStr=fixdt(0, 11, 0)  PortDimensions=1  SampleTime=6.66666666666667e-09
  Simple Dual Port RAM : hdlsllib/HDL RAMs/Simple Dual Port RAM  ram_size=ceil(log2(maxRho*2))
      settings: SourceProductName=Simulink  SourceProductBaseCode=SL
  rd_data : Outport
  wires:
  rd_addr/1 -> Simple Dual Port RAM/4
  wr_en/1 -> Simple Dual Port RAM/3
  wr_addr/1 -> Simple Dual Port RAM/2
  wr_data/1 -> Simple Dual Port RAM/1
  Simple Dual Port RAM/1 -> rd_data/1

== system gm_parallel_lht/Parallel LHT/Parallel LHT Accumulator/Accumulator with Switches/Accumulator_instance22/Block RAM/Simple Dual Port RAM ==
  wr_data : Inport  OutDataTypeStr=fixdt(0, 11, 0)  PortDimensions=1  SampleTime=6.66666666666667e-09
  wr_addr : Inport  Port=2  OutDataTypeStr=fixdt(0, 11, 0)  PortDimensions=1  SampleTime=6.66666666666667e-09
  wr_en : Inport  Port=3  OutDataTypeStr=boolean  PortDimensions=1  SampleTime=6.66666666666667e-09
  rd_addr : Inport  Port=4  OutDataTypeStr=fixdt(0, 11, 0)  PortDimensions=1  SampleTime=6.66666666666667e-09
  Simple Dual Port RAM : hdlsllib/HDL RAMs/Simple Dual Port RAM  ram_size=ceil(log2(maxRho*2))
      settings: SourceProductName=Simulink  SourceProductBaseCode=SL
  rd_data : Outport
  wires:
  rd_addr/1 -> Simple Dual Port RAM/4
  wr_en/1 -> Simple Dual Port RAM/3
  wr_addr/1 -> Simple Dual Port RAM/2
  wr_data/1 -> Simple Dual Port RAM/1
  Simple Dual Port RAM/1 -> rd_data/1

== system gm_parallel_lht/Parallel LHT/Parallel LHT Accumulator/Accumulator with Switches/Accumulator_instance23/Block RAM/Simple Dual Port RAM ==
  wr_data : Inport  OutDataTypeStr=fixdt(0, 11, 0)  PortDimensions=1  SampleTime=6.66666666666667e-09
  wr_addr : Inport  Port=2  OutDataTypeStr=fixdt(0, 11, 0)  PortDimensions=1  SampleTime=6.66666666666667e-09
  wr_en : Inport  Port=3  OutDataTypeStr=boolean  PortDimensions=1  SampleTime=6.66666666666667e-09
  rd_addr : Inport  Port=4  OutDataTypeStr=fixdt(0, 11, 0)  PortDimensions=1  SampleTime=6.66666666666667e-09
  Simple Dual Port RAM : hdlsllib/HDL RAMs/Simple Dual Port RAM  ram_size=ceil(log2(maxRho*2))
      settings: SourceProductName=Simulink  SourceProductBaseCode=SL
  rd_data : Outport
  wires:
  rd_addr/1 -> Simple Dual Port RAM/4
  wr_en/1 -> Simple Dual Port RAM/3
  wr_addr/1 -> Simple Dual Port RAM/2
  wr_data/1 -> Simple Dual Port RAM/1
  Simple Dual Port RAM/1 -> rd_data/1

== system gm_parallel_lht/Parallel LHT/Parallel LHT Accumulator/Accumulator with Switches/Accumulator_instance24/Block RAM/Simple Dual Port RAM ==
  wr_data : Inport  OutDataTypeStr=fixdt(0, 11, 0)  PortDimensions=1  SampleTime=6.66666666666667e-09
  wr_addr : Inport  Port=2  OutDataTypeStr=fixdt(0, 11, 0)  PortDimensions=1  SampleTime=6.66666666666667e-09
  wr_en : Inport  Port=3  OutDataTypeStr=boolean  PortDimensions=1  SampleTime=6.66666666666667e-09
  rd_addr : Inport  Port=4  OutDataTypeStr=fixdt(0, 11, 0)  PortDimensions=1  SampleTime=6.66666666666667e-09
  Simple Dual Port RAM : hdlsllib/HDL RAMs/Simple Dual Port RAM  ram_size=ceil(log2(maxRho*2))
      settings: SourceProductName=Simulink  SourceProductBaseCode=SL
  rd_data : Outport
  wires:
  rd_addr/1 -> Simple Dual Port RAM/4
  wr_en/1 -> Simple Dual Port RAM/3
  wr_addr/1 -> Simple Dual Port RAM/2
  wr_data/1 -> Simple Dual Port RAM/1
  Simple Dual Port RAM/1 -> rd_data/1

== system gm_parallel_lht/Parallel LHT/Parallel LHT Accumulator/Accumulator with Switches/Accumulator_instance25/Block RAM/Simple Dual Port RAM ==
  wr_data : Inport  OutDataTypeStr=fixdt(0, 11, 0)  PortDimensions=1  SampleTime=6.66666666666667e-09
  wr_addr : Inport  Port=2  OutDataTypeStr=fixdt(0, 11, 0)  PortDimensions=1  SampleTime=6.66666666666667e-09
  wr_en : Inport  Port=3  OutDataTypeStr=boolean  PortDimensions=1  SampleTime=6.66666666666667e-09
  rd_addr : Inport  Port=4  OutDataTypeStr=fixdt(0, 11, 0)  PortDimensions=1  SampleTime=6.66666666666667e-09
  Simple Dual Port RAM : hdlsllib/HDL RAMs/Simple Dual Port RAM  ram_size=ceil(log2(maxRho*2))
      settings: SourceProductName=Simulink  SourceProductBaseCode=SL
  rd_data : Outport
  wires:
  rd_addr/1 -> Simple Dual Port RAM/4
  wr_en/1 -> Simple Dual Port RAM/3
  wr_addr/1 -> Simple Dual Port RAM/2
  wr_data/1 -> Simple Dual Port RAM/1
  Simple Dual Port RAM/1 -> rd_data/1

== system gm_parallel_lht/Parallel LHT/Parallel LHT Accumulator/Accumulator with Switches/Accumulator_instance26/Block RAM/Simple Dual Port RAM ==
  wr_data : Inport  OutDataTypeStr=fixdt(0, 11, 0)  PortDimensions=1  SampleTime=6.66666666666667e-09
  wr_addr : Inport  Port=2  OutDataTypeStr=fixdt(0, 11, 0)  PortDimensions=1  SampleTime=6.66666666666667e-09
  wr_en : Inport  Port=3  OutDataTypeStr=boolean  PortDimensions=1  SampleTime=6.66666666666667e-09
  rd_addr : Inport  Port=4  OutDataTypeStr=fixdt(0, 11, 0)  PortDimensions=1  SampleTime=6.66666666666667e-09
  Simple Dual Port RAM : hdlsllib/HDL RAMs/Simple Dual Port RAM  ram_size=ceil(log2(maxRho*2))
      settings: SourceProductName=Simulink  SourceProductBaseCode=SL
  rd_data : Outport
  wires:
  rd_addr/1 -> Simple Dual Port RAM/4
  wr_en/1 -> Simple Dual Port RAM/3
  wr_addr/1 -> Simple Dual Port RAM/2
  wr_data/1 -> Simple Dual Port RAM/1
  Simple Dual Port RAM/1 -> rd_data/1

== system gm_parallel_lht/Parallel LHT/Parallel LHT Accumulator/Accumulator with Switches/Accumulator_instance27/Block RAM/Simple Dual Port RAM ==
  wr_data : Inport  OutDataTypeStr=fixdt(0, 11, 0)  PortDimensions=1  SampleTime=6.66666666666667e-09
  wr_addr : Inport  Port=2  OutDataTypeStr=fixdt(0, 11, 0)  PortDimensions=1  SampleTime=6.66666666666667e-09
  wr_en : Inport  Port=3  OutDataTypeStr=boolean  PortDimensions=1  SampleTime=6.66666666666667e-09
  rd_addr : Inport  Port=4  OutDataTypeStr=fixdt(0, 11, 0)  PortDimensions=1  SampleTime=6.66666666666667e-09
  Simple Dual Port RAM : hdlsllib/HDL RAMs/Simple Dual Port RAM  ram_size=ceil(log2(maxRho*2))
      settings: SourceProductName=Simulink  SourceProductBaseCode=SL
  rd_data : Outport
  wires:
  rd_addr/1 -> Simple Dual Port RAM/4
  wr_en/1 -> Simple Dual Port RAM/3
  wr_addr/1 -> Simple Dual Port RAM/2
  wr_data/1 -> Simple Dual Port RAM/1
  Simple Dual Port RAM/1 -> rd_data/1

== system gm_parallel_lht/Parallel LHT/Parallel LHT Accumulator/Accumulator with Switches/Accumulator_instance28/Block RAM/Simple Dual Port RAM ==
  wr_data : Inport  OutDataTypeStr=fixdt(0, 11, 0)  PortDimensions=1  SampleTime=6.66666666666667e-09
  wr_addr : Inport  Port=2  OutDataTypeStr=fixdt(0, 11, 0)  PortDimensions=1  SampleTime=6.66666666666667e-09
  wr_en : Inport  Port=3  OutDataTypeStr=boolean  PortDimensions=1  SampleTime=6.66666666666667e-09
  rd_addr : Inport  Port=4  OutDataTypeStr=fixdt(0, 11, 0)  PortDimensions=1  SampleTime=6.66666666666667e-09
  Simple Dual Port RAM : hdlsllib/HDL RAMs/Simple Dual Port RAM  ram_size=ceil(log2(maxRho*2))
      settings: SourceProductName=Simulink  SourceProductBaseCode=SL
  rd_data : Outport
  wires:
  rd_addr/1 -> Simple Dual Port RAM/4
  wr_en/1 -> Simple Dual Port RAM/3
  wr_addr/1 -> Simple Dual Port RAM/2
  wr_data/1 -> Simple Dual Port RAM/1
  Simple Dual Port RAM/1 -> rd_data/1

== system gm_parallel_lht/Parallel LHT/Parallel LHT Accumulator/Accumulator with Switches/Accumulator_instance29/Block RAM/Simple Dual Port RAM ==
  wr_data : Inport  OutDataTypeStr=fixdt(0, 11, 0)  PortDimensions=1  SampleTime=6.66666666666667e-09
  wr_addr : Inport  Port=2  OutDataTypeStr=fixdt(0, 11, 0)  PortDimensions=1  SampleTime=6.66666666666667e-09
  wr_en : Inport  Port=3  OutDataTypeStr=boolean  PortDimensions=1  SampleTime=6.66666666666667e-09
  rd_addr : Inport  Port=4  OutDataTypeStr=fixdt(0, 11, 0)  PortDimensions=1  SampleTime=6.66666666666667e-09
  Simple Dual Port RAM : hdlsllib/HDL RAMs/Simple Dual Port RAM  ram_size=ceil(log2(maxRho*2))
      settings: SourceProductName=Simulink  SourceProductBaseCode=SL
  rd_data : Outport
  wires:
  rd_addr/1 -> Simple Dual Port RAM/4
  wr_en/1 -> Simple Dual Port RAM/3
  wr_addr/1 -> Simple Dual Port RAM/2
  wr_data/1 -> Simple Dual Port RAM/1
  Simple Dual Port RAM/1 -> rd_data/1

== system gm_parallel_lht/Parallel LHT/Parallel LHT Accumulator/Accumulator with Switches/Accumulator_instance3/Block RAM/Simple Dual Port RAM ==
  wr_data : Inport  OutDataTypeStr=fixdt(0, 11, 0)  PortDimensions=1  SampleTime=6.66666666666667e-09
  wr_addr : Inport  Port=2  OutDataTypeStr=fixdt(0, 11, 0)  PortDimensions=1  SampleTime=6.66666666666667e-09
  wr_en : Inport  Port=3  OutDataTypeStr=boolean  PortDimensions=1  SampleTime=6.66666666666667e-09
  rd_addr : Inport  Port=4  OutDataTypeStr=fixdt(0, 11, 0)  PortDimensions=1  SampleTime=6.66666666666667e-09
  Simple Dual Port RAM : hdlsllib/HDL RAMs/Simple Dual Port RAM  ram_size=ceil(log2(maxRho*2))
      settings: SourceProductName=Simulink  SourceProductBaseCode=SL
  rd_data : Outport
  wires:
  rd_addr/1 -> Simple Dual Port RAM/4
  wr_en/1 -> Simple Dual Port RAM/3
  wr_addr/1 -> Simple Dual Port RAM/2
  wr_data/1 -> Simple Dual Port RAM/1
  Simple Dual Port RAM/1 -> rd_data/1

== system gm_parallel_lht/Parallel LHT/Parallel LHT Accumulator/Accumulator with Switches/Accumulator_instance30/Block RAM/Simple Dual Port RAM ==
  wr_data : Inport  OutDataTypeStr=fixdt(0, 11, 0)  PortDimensions=1  SampleTime=6.66666666666667e-09
  wr_addr : Inport  Port=2  OutDataTypeStr=fixdt(0, 11, 0)  PortDimensions=1  SampleTime=6.66666666666667e-09
  wr_en : Inport  Port=3  OutDataTypeStr=boolean  PortDimensions=1  SampleTime=6.66666666666667e-09
  rd_addr : Inport  Port=4  OutDataTypeStr=fixdt(0, 11, 0)  PortDimensions=1  SampleTime=6.66666666666667e-09
  Simple Dual Port RAM : hdlsllib/HDL RAMs/Simple Dual Port RAM  ram_size=ceil(log2(maxRho*2))
      settings: SourceProductName=Simulink  SourceProductBaseCode=SL
  rd_data : Outport
  wires:
  rd_addr/1 -> Simple Dual Port RAM/4
  wr_en/1 -> Simple Dual Port RAM/3
  wr_addr/1 -> Simple Dual Port RAM/2
  wr_data/1 -> Simple Dual Port RAM/1
  Simple Dual Port RAM/1 -> rd_data/1

== system gm_parallel_lht/Parallel LHT/Parallel LHT Accumulator/Accumulator with Switches/Accumulator_instance31/Block RAM/Simple Dual Port RAM ==
  wr_data : Inport  OutDataTypeStr=fixdt(0, 11, 0)  PortDimensions=1  SampleTime=6.66666666666667e-09
  wr_addr : Inport  Port=2  OutDataTypeStr=fixdt(0, 11, 0)  PortDimensions=1  SampleTime=6.66666666666667e-09
  wr_en : Inport  Port=3  OutDataTypeStr=boolean  PortDimensions=1  SampleTime=6.66666666666667e-09
  rd_addr : Inport  Port=4  OutDataTypeStr=fixdt(0, 11, 0)  PortDimensions=1  SampleTime=6.66666666666667e-09
  Simple Dual Port RAM : hdlsllib/HDL RAMs/Simple Dual Port RAM  ram_size=ceil(log2(maxRho*2))
      settings: SourceProductName=Simulink  SourceProductBaseCode=SL
  rd_data : Outport
  wires:
  rd_addr/1 -> Simple Dual Port RAM/4
  wr_en/1 -> Simple Dual Port RAM/3
  wr_addr/1 -> Simple Dual Port RAM/2
  wr_data/1 -> Simple Dual Port RAM/1
  Simple Dual Port RAM/1 -> rd_data/1

== system gm_parallel_lht/Parallel LHT/Parallel LHT Accumulator/Accumulator with Switches/Accumulator_instance32/Block RAM/Simple Dual Port RAM ==
  wr_data : Inport  OutDataTypeStr=fixdt(0, 11, 0)  PortDimensions=1  SampleTime=6.66666666666667e-09
  wr_addr : Inport  Port=2  OutDataTypeStr=fixdt(0, 11, 0)  PortDimensions=1  SampleTime=6.66666666666667e-09
  wr_en : Inport  Port=3  OutDataTypeStr=boolean  PortDimensions=1  SampleTime=6.66666666666667e-09
  rd_addr : Inport  Port=4  OutDataTypeStr=fixdt(0, 11, 0)  PortDimensions=1  SampleTime=6.66666666666667e-09
  Simple Dual Port RAM : hdlsllib/HDL RAMs/Simple Dual Port RAM  ram_size=ceil(log2(maxRho*2))
      settings: SourceProductName=Simulink  SourceProductBaseCode=SL
  rd_data : Outport
  wires:
  rd_addr/1 -> Simple Dual Port RAM/4
  wr_en/1 -> Simple Dual Port RAM/3
  wr_addr/1 -> Simple Dual Port RAM/2
  wr_data/1 -> Simple Dual Port RAM/1
  Simple Dual Port RAM/1 -> rd_data/1

== system gm_parallel_lht/Parallel LHT/Parallel LHT Accumulator/Accumulator with Switches/Accumulator_instance33/Block RAM/Simple Dual Port RAM ==
  wr_data : Inport  OutDataTypeStr=fixdt(0, 11, 0)  PortDimensions=1  SampleTime=6.66666666666667e-09
  wr_addr : Inport  Port=2  OutDataTypeStr=fixdt(0, 11, 0)  PortDimensions=1  SampleTime=6.66666666666667e-09
  wr_en : Inport  Port=3  OutDataTypeStr=boolean  PortDimensions=1  SampleTime=6.66666666666667e-09
  rd_addr : Inport  Port=4  OutDataTypeStr=fixdt(0, 11, 0)  PortDimensions=1  SampleTime=6.66666666666667e-09
  Simple Dual Port RAM : hdlsllib/HDL RAMs/Simple Dual Port RAM  ram_size=ceil(log2(maxRho*2))
      settings: SourceProductName=Simulink  SourceProductBaseCode=SL
  rd_data : Outport
  wires:
  rd_addr/1 -> Simple Dual Port RAM/4
  wr_en/1 -> Simple Dual Port RAM/3
  wr_addr/1 -> Simple Dual Port RAM/2
  wr_data/1 -> Simple Dual Port RAM/1
  Simple Dual Port RAM/1 -> rd_data/1

== system gm_parallel_lht/Parallel LHT/Parallel LHT Accumulator/Accumulator with Switches/Accumulator_instance34/Block RAM/Simple Dual Port RAM ==
  wr_data : Inport  OutDataTypeStr=fixdt(0, 11, 0)  PortDimensions=1  SampleTime=6.66666666666667e-09
  wr_addr : Inport  Port=2  OutDataTypeStr=fixdt(0, 11, 0)  PortDimensions=1  SampleTime=6.66666666666667e-09
  wr_en : Inport  Port=3  OutDataTypeStr=boolean  PortDimensions=1  SampleTime=6.66666666666667e-09
  rd_addr : Inport  Port=4  OutDataTypeStr=fixdt(0, 11, 0)  PortDimensions=1  SampleTime=6.66666666666667e-09
  Simple Dual Port RAM : hdlsllib/HDL RAMs/Simple Dual Port RAM  ram_size=ceil(log2(maxRho*2))
      settings: SourceProductName=Simulink  SourceProductBaseCode=SL
  rd_data : Outport
  wires:
  rd_addr/1 -> Simple Dual Port RAM/4
  wr_en/1 -> Simple Dual Port RAM/3
  wr_addr/1 -> Simple Dual Port RAM/2
  wr_data/1 -> Simple Dual Port RAM/1
  Simple Dual Port RAM/1 -> rd_data/1
